simulink model "h"  (R2016a)
settings: Solver=VariableStepAuto  StartTime=0.0  StopTime=10.0  RelTol=1e-3
undefined symbols (not defined in the file): A, a1, a2, A3, A3A4, A4, b1, b2, beta, c1, c2, Cppx, Cppy, Cpx, Cpy, FM, Fs, M, m, R1, R2, R4, R5, RL, s, V4, V5, V5m, VA, VB, W_n1, yita_n1
settings Model: Creator=xlh  LastModifiedBy=xlh

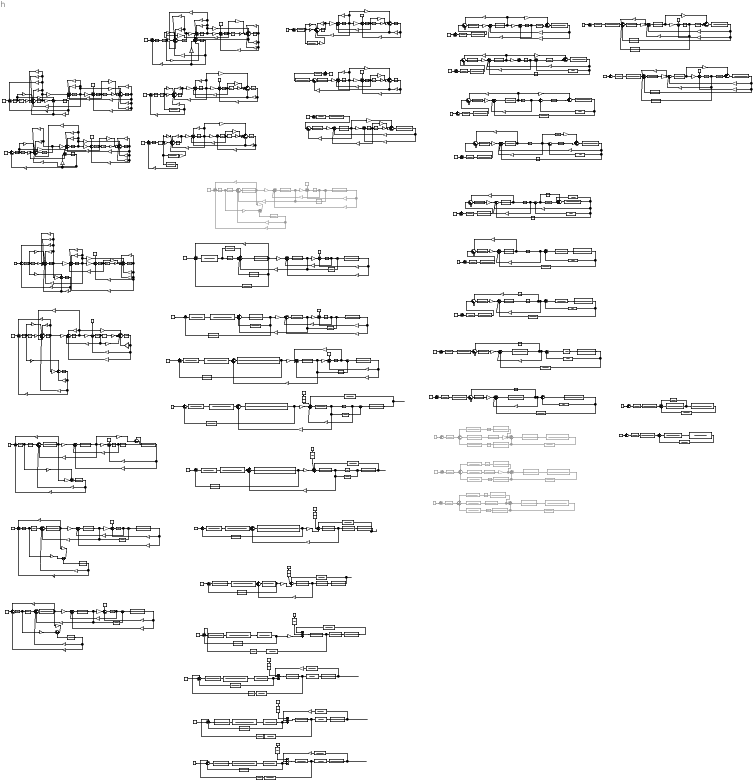
== system h ==
  note: 1.86e3rad/s
      | 296Hz
  note: 合并相同通道
  note: 合并相同通道
  note: y合并
  note: P4 合并
  note: V5-V4等式
  note: 忽略VB/beta
  note: 第三次化简P4
  note: 忽略, Cpx=3.3,远大于其他项，在频率为几赫兹时
  note: 忽略
  note: yita_n1=0.4725 W_n1=74081rad/s
  note: 第一次简化P5
  note: PB
  note: PB
  note: PB
  note: PB
  note: PB
  note: PB
  note: PB
  note: PB
  note: PB
  note: PB
  note: PB
  note: PB
  note: PB
  note: 第二次简化Vx
  note: PB
  note: 忽略
  note: yita_n1=0.4725 W_n1=74081rad/s
  note: PB
  note: 忽略
  note: yita_n1=0.4725 W_n1=74081rad/s
  note: PB
  note: 忽略, Cpx=3.3,远大于其他项，在频率为几赫兹时
  note: 忽略
  note: yita_n1=0.4725 W_n1=74081rad/s
  note: PB
  note: 忽略, Cpx=3.3,远大于其他项，在频率为几赫兹时
  note: 忽略
  note: yita_n1=0.4725 W_n1=74081rad/s
  note: PB
  note: PB
  note: PB
  note: PB
  note: PB
  note: PB
  note: PB
  note: 反馈通道合并
  note: PB
  note: x合并
  note: PB
  note: 挪动Vx',Vx'' = PA*A4/(Ms)-Vx'
  note: PB
  note: 合并
  note: PB
  note: x合并
  note: PB
  note: x合并
  note: PB
  note: Vx'''=-Vx''
  note: PB
  note: move branch
  note: PB
  note: merge
  note: PB
  note: move PB
  note: PB
  note: merge
  note: PB
  note: move
  note: PB
  note: simplify
  note: PB
  note: simplify
  note: PB
  note: move and merge
  note: PB
  note: 3.24e4rad/s
      | 5156Hz
      | 固定阻尼1.3747
  note: 1.86e3rad/s
      | 296Hz
  note: move
  note: PB
  note: 3.24e4rad/s
      | 5156Hz
      | 固定阻尼1.3747
  note: 合并相同通道
  note: desire frequent :1-10Hz
  note: move branch
  note: merge
  note: PB
  note: desire frequent :1-10Hz
  {1..5,8} (6 alike) : TransferFcn  Numerator=[A*R4*V5/beta (-Cpy*R4/V5)*beta -Cpy]  Denominator=[R4*V5/beta 1 0]
  {9..10,14..16,18..19,21,23..24,67..68} (12 alike) : Gain  Gain=1/R1
  17 : Gain  Gain=A4
  20 : Gain  Gain=A4
  6 : TransferFcn  Numerator=[A*R4*V5/beta (2*A+Cpy*R4*R5/beta) Cpy]  Denominator=[R4*V5/beta 1 0]
  7 : TransferFcn  Numerator=[A*R4*V5/beta (2*A+Cpy*R4*R5/beta) Cpy]  Denominator=[R4*V5/beta 1 0]
  95 : Gain  Gain=A4
  C3 : Constant  Value=Fs
  C4 : Constant  Value=Fs
  Constant{,2,4,6,8,10,14,16,18,20,22,24,26,28,30,32,34,36,38,40..42,44,46,48,50..59,64..65} (37 alike) : Constant  Value=FM
  Constant{1,3,5,7,9,11,15,17,19,21,23,25,27,29,31,33,35,37,39,43,45,47} (22 alike) : Constant  Value=Fs
  Constant{12,61..63} (4 alike) : Constant  Commented=on  Value=FM
  Constant13 : Constant  Commented=on  Value=Fs
  Gain{,20,44,142..143,165,193,208,229} (9 alike) : Gain  Gain=Cpy
  Gain{1,11..12,21,23..24,45,47..48,53,55,65,68,87,89,145,155,168,194,210} (20 alike) : Gain  Gain=1/R4
  Gain{10,22,144,209} (4 alike) : Gain  Gain=Cppy
  Gain100 : Gain  Commented=on  Gain=1/R4
  Gain101 : Gain  Commented=on  Gain=A4
  Gain{102,106,286..287} (4 alike) : Gain  Commented=on  Gain=1/R2
  Gain103 : Gain  Commented=on  Gain=A
  Gain104 : Gain  Commented=on  Gain=A3
  Gain105 : Gain  Commented=on  Gain=A
  Gain107 : Gain  Commented=on  Gain=A3
  Gain108 : Gain  Commented=on  Gain=A
  Gain109 : Gain  Commented=on  Gain=1/R1
  Gain{16,18,28,30,52,54,69,71,90,110,113,116,150,152,173..176,198..199,215,217,238..239,246..247} (26 alike) : Gain  Gain=A4
  Gain{2,7..8,14,26,32,37..38,56,61,70,72,76,84,91,95,111,114,118,120..121,125,129..132,134..138,148,154,159..161,177,182,185,190,195,200,204..205,213,219,223..225,240,244..245,249,254,261,265..267,270..271,273..274,276..277,279..280,282..283,285} (69 alike) : Gain  Gain=1/R2
  Gain{4,34,41,50,58,62,74,77,82,85,93,96,112,115,119,122..123,126,133,156,158,178,180..181,186,188..189,201,203,220,222,235,241,243,250,252..253,262..264,268..269,272,275,278,281,284,288} (48 alike) : Gain  Gain=A3
  Gain{13,15,25,27,42..43,66..67,80..81,88,98,117,127..128,147,149,192,212,214,231..234,248,255..258,260} (30 alike) : Gain  Gain=1/R1
  Gain{3,6,9,33,36,39..40,57,60,63..64,73,75,78..79,83,86,92,94,97,124,146,162,166,169,211,259} (27 alike) : Gain  Gain=A
  Gain139 : Gain  Gain=R2
  Gain140 : Gain  Gain=R2
  Gain141 : Gain  Gain=R2
  Gain{17,29,151,216} (4 alike) : Gain  Gain=1/RL
  Gain{19,31,153,218} (4 alike) : Gain  Gain=Cppx
  Gain{5,35,59,157,179,187,202,221,242,251} (10 alike) : Gain  Gain=Cpx
  Gain163 : Gain  Gain=2*A
  Gain164 : Gain  Gain=2/R4
  Gain{49,167,170,196,236} (5 alike) : Gain  Gain=1/R1+1/R2
  Gain{51,171..172,197,237} (5 alike) : Gain  Gain=1/R1+1/RL+Cppx
  Gain183 : Gain  Gain=1/R2+Cppy
  Gain{184,207,226,230} (4 alike) : Gain  Gain=A*s
  Gain191 : Gain  Gain=1/R2+Cppy
  Gain206 : Gain  Gain=1/R2+Cppy
  Gain227 : Gain  Gain=2*A*s
  Gain228 : Gain  Gain=2/R4
  Gain46 : Gain  Gain=Cppy+1/R4+1/R2
  Gain99 : Gain  Commented=on  Gain=1/R4
  Sum{,6,14,20,26,31,43,49,51,57..58,65,68,71..72,75,77,79,85,87,95,100,106,111,116,121,127,130,137,142,147,152,155,160,164,176..177} (37 alike) : Sum  Inputs=+--
  Sum{1,7,15,21,27,32,80,86,91,96,101} (11 alike) : Sum  Inputs=-----++
  Sum{4,10,12,18,24..25,42,47..48,83,89,93,98,104,109,114,119,126,135,140} (20 alike) : Sum  Inputs=--+
  Sum102 : Sum  Inputs=++-+
  Sum{3,9,17,23,29,34,45,52,55,82,88,92,97,103,108,113,118,134,139} (19 alike) : Sum  Inputs=--+++
  Sum{5,11,13,84,90,94,99,105,110,115,120,125,131,136,141,145} (16 alike) : Sum  Inputs=+-----
  Sum{64,107,112,117,122,128,143,148,153,157} (10 alike) : Sum  Inputs=|++
  Sum{123,129,144,149,154,158,162,166} (8 alike) : Sum  Inputs=--+-++
  Sum{67,70,73..74,76,78,124,163,178..180} (11 alike) : Sum  Inputs=+++
  Sum132 : Sum  Inputs=+-+
  Sum133 : Sum  Inputs=|++++
  Sum138 : Sum  Inputs=|++++
  Sum{30,35,46,53,56,61,146,151} (8 alike) : Sum  Inputs=|-+
  Sum150 : Sum  Inputs=------
  Sum156 : Sum  Inputs=+-+
  Sum{2,8,16,22,159} (5 alike) : Sum  Inputs=++-
  Sum161 : Sum  Inputs=|+-
  Sum165 : Sum  Inputs=|+-
  Sum{37,167..168,172} (4 alike) : Sum  Commented=on  Inputs=+--
  Sum{169..171,173..175} (6 alike) : Sum  Commented=on  Inputs=+++
  Sum19 : Sum  Inputs=+-
  Sum28 : Sum
  Sum33 : Sum
  Sum36 : Sum  Commented=on  Inputs=--+
  Sum38 : Sum  Commented=on  Inputs=-----++
  Sum39 : Sum  Commented=on
  Sum40 : Sum  Commented=on  Inputs=--+++
  Sum41 : Sum  Commented=on  Inputs=|-+
  Sum{44,54,59,62,66,69} (6 alike) : Sum  Inputs=+--+-++
  Sum50 : Sum  Inputs=+----++
  Sum60 : Sum  Inputs=+++++
  Sum63 : Sum  Inputs=+++++
  Sum81 : Sum  Inputs=++-+
  T1 : TransferFcn  Numerator=[M 0]  Denominator=[A3*R2]
  Tra : TransferFcn  Numerator=[beta]  Denominator=[V4 0]
  Transfer Fcn{,8,22,30,38,45,149,157,165,183} (10 alike) : TransferFcn  Denominator=[m 0]
  Transfer Fcn{1,7,9,15,21,23,150,156,158,164,166,172,181,184,190,194,201} (17 alike) : TransferFcn  Denominator=[1 0]
  Transfer Fcn{2,10,16,159,167,176,185} (7 alike) : TransferFcn  Numerator=[beta]  Denominator=[V4 0]
  Transfer Fcn{88,100,103,113} (4 alike) : TransferFcn  Denominator=[(VB/beta+M) 1/R1+1/R2]
  Transfer Fcn{35,43,59,69,78,86,93,101,107,114} (10 alike) : TransferFcn  Numerator=[A4 Cpx]  Denominator="[VA/beta  (1/R1+1/RL+Cppx) 0]"
  Transfer Fcn102 : TransferFcn  Numerator="[A3A4  (M/R1+A3*Cpx)]"  Denominator=[A4*M M*Cpx 0]
  Transfer Fcn{64,71,82,90,96,104} (6 alike) : TransferFcn  Numerator=[V5/beta 1/R4]  Denominator=[V5m/beta m/R4 A^2]
  Transfer Fcn{91,97,105,110,117,126,135,144,151,268,272,280,286,323,326} (15 alike) : TransferFcn  Numerator=[M/R1 A3*A4]  Denominator=[M 0]
  Transfer Fcn{6,14,20,28,36,44,60,70,79,92,98,106,111,118,155,163,171,180,189,193,200,206,211,227,235} (25 alike) : TransferFcn  Denominator=[M 0]
  Transfer Fcn108 : TransferFcn  Numerator="[A3A4  (M/R1+A3*Cpx)]"  Denominator=[A4*M M*Cpx 0]
  Transfer Fcn{109,116,125,134,143} (5 alike) : TransferFcn  Numerator=[1/m beta/(R4*V5*m)]  Denominator=[1 2*yita_n1*W_n1 W_n1^2]
  Transfer Fcn{3,11,17,152,186} (5 alike) : TransferFcn  Numerator=[beta]  Denominator=[V5 0]
  Transfer Fcn{57,76,83..84,99,112,119,128,137,146} (10 alike) : TransferFcn  Numerator=[-A*R4*V5/beta 0]  Denominator=[R4*V5/beta 1]
  Transfer Fcn115 : TransferFcn  Numerator="[A3A4  (M/R1+A3*Cpx)]"  Denominator=[A4*M M*Cpx 0]
  Transfer Fcn{4,12,18,153,161,169,178,187,191} (9 alike) : TransferFcn  Numerator=[beta]  Denominator=[VB 0]
  Transfer Fcn{120,129,138,147} (4 alike) : TransferFcn  Numerator=[A*beta^2 0]  Denominator=[R4*V5 beta]
  Transfer Fcn{121,130,139,148} (4 alike) : TransferFcn  Denominator=[R2*V4 0]
  Transfer Fcn122 : TransferFcn  Denominator=[(VB/beta+M)*R2 R2/R1+1]
  Transfer Fcn123 : TransferFcn  Numerator=[Cpx]  Denominator="[VA/beta  (1/R1+1/RL+Cppx) 0]"
  Transfer Fcn124 : TransferFcn  Numerator=[(A3*Cpx)]  Denominator=[M*Cpx 0]
  Transfer Fcn127 : TransferFcn  Numerator=[R2]  Denominator=[M 0]
  Transfer Fcn{5,13,19,154,162,170,179,188,192} (9 alike) : TransferFcn  Numerator=[beta]  Denominator=[VA 0]
  Transfer Fcn131 : TransferFcn  Denominator=[M*R2 R2/R1+1]
  Transfer Fcn132 : TransferFcn  Numerator=[Cpx]  Denominator="[VA/beta  (1/R1+1/RL+Cppx) 0]"
  Transfer Fcn133 : TransferFcn  Numerator=[(A3*Cpx)]  Denominator=[M*Cpx 0]
  Transfer Fcn136 : TransferFcn  Numerator=[R2]  Denominator=[M 0]
  Transfer Fcn140 : TransferFcn  Denominator=[(VB/beta+M)*R2 R2/R1+1]
  Transfer Fcn141 : TransferFcn  Numerator=[Cpx]  Denominator="[VA/beta  (1/R1+1/RL+Cppx) 0]"
  Transfer Fcn142 : TransferFcn  Numerator=[(A3*Cpx)]  Denominator=[M*Cpx 0]
  Transfer Fcn145 : TransferFcn  Numerator=[R2]  Denominator=[M 0]
  Transfer Fcn{160,168,173,182} (4 alike) : TransferFcn  Numerator=[2*A Cpy]  Denominator=[V5/beta 2/R4]
  Transfer Fcn174 : TransferFcn  Denominator=[a1 b1 c1]
  Transfer Fcn175 : TransferFcn  Denominator=[a1 b1 c1]
  Transfer Fcn{177,197,199,204,217,223..225,233,241,250,261,274} (13 alike) : TransferFcn  Denominator=[V4/beta 1/R2+Cppy]
  Transfer Fcn{195,202,208,213,221,229,237,245,254,265,270,278,284} (13 alike) : TransferFcn  Numerator=[-V5*A/beta/R4 2*A Cpy]  Denominator=[V5/beta/R4 2/R4^2]
  Transfer Fcn196 : TransferFcn  Denominator=[a1 b1 c1]
  Transfer Fcn{27,198,205,210,218,226,234,242,251} (9 alike) : TransferFcn  Denominator=[VA/beta 1/R1+1/RL+Cppx]
  Transfer Fcn{26,34,42,58,68,77,85,203,209,214,222,230,238,246,255,266,271} (17 alike) : TransferFcn  Denominator=[VB/beta 1/R1+1/R2]
  Transfer Fcn{29,207,212,220,228,236,244,253} (8 alike) : TransferFcn  Numerator=[A4 Cpx]  Denominator=[1 0]
  Transfer Fcn{215,256,259..260,327,329..330,332} (8 alike) : TransferFcn  Numerator=[A4]  Denominator=[M 0]
  Transfer Fcn216 : TransferFcn  Numerator=[A3*A4]  Denominator=[M 0]
  Transfer Fcn{94,219,243,252,263,267} (6 alike) : TransferFcn  Numerator=[A3]  Denominator=[M 0]
  Transfer Fcn231 : TransferFcn  Numerator=[A3/R2]  Denominator=[VB/beta 1/R1+1/R2]
  Transfer Fcn232 : TransferFcn  Numerator=[1/R2*R1]  Denominator=[VB/beta 1/R1+1/R2]
  Transfer Fcn239 : TransferFcn  Numerator=[A3/R2]  Denominator=[VB/beta 1/R1+1/R2]
  Transfer Fcn{24,32,37,56,66} (5 alike) : TransferFcn  Denominator=[V4/beta Cppy+1/R4+1/R2]
  Transfer Fcn240 : TransferFcn  Numerator=[1/R2*R1]  Denominator=[VB/beta 1/R1+1/R2]
  Transfer Fcn247 : TransferFcn  Denominator=[(VA/beta) 1/R1+1/RL+Cppx+A4/A3/R1]
  Transfer Fcn248 : TransferFcn  Numerator=[A3*A4]  Denominator=[M 0]
  Transfer Fcn249 : TransferFcn  Numerator=[M 0]  Denominator=[A3]
  Transfer Fcn25 : TransferFcn  Denominator=[V5/beta 1/R4]
  Transfer Fcn257 : TransferFcn  Numerator=[A3*A4]  Denominator=[M 0]
  Transfer Fcn258 : TransferFcn  Numerator=[M 0]  Denominator=[A3*R1]
  Transfer Fcn262 : TransferFcn  Denominator=[(VA/beta) 1/R1+1/RL+Cppx+A4/A3/R1]
  Transfer Fcn264 : TransferFcn  Numerator=[-M/A3/R1 -A4 -Cpx]  Denominator=[1 0]
  Transfer Fcn269 : TransferFcn  Numerator=[M/A3/R1 A4 Cpx]  Denominator=[1 0]
  Transfer Fcn273 : TransferFcn  Numerator=[M 0]  Denominator=[A3]
  Transfer Fcn275 : TransferFcn  Denominator=[(VA/beta) 1/R1+1/RL+Cppx+A4/A3/R1]
  Transfer Fcn276 : TransferFcn  Numerator=[Cpx]  Denominator=[(VA/beta) 1/R1+1/RL+Cppx+A4/A3/R1 0]
  Transfer Fcn277 : TransferFcn  Numerator=[Cpx]  Denominator=[1 0]
  Transfer Fcn279 : TransferFcn  Numerator=[A3]  Denominator=[M*VB/beta M/R1+M/R2 0]
  Transfer Fcn281 : TransferFcn  Numerator=[M 0]  Denominator=[A3*R2]
  Transfer Fcn283 : TransferFcn  Commented=on  Denominator=[V4/beta 1/R2+Cppy]
  Transfer Fcn285 : TransferFcn  Numerator=[A3]  Denominator=[M*VB/beta M/R1+M/R2 0]
  Transfer Fcn287 : TransferFcn  Numerator=[-M/A3/R1 -A4 -Cpx]  Denominator=[(VA/beta) A4^2 Cpx*A4]
  Transfer Fcn288 : TransferFcn  Commented=on  Numerator=[M/A3/R1 A4 Cpx]  Denominator=[(VA/beta+2*M*A4/A3/R1) A4^2 Cpx*A4]
  Transfer Fcn289 : TransferFcn  Commented=on  Numerator=[-V5*A/beta/R4 2*A Cpy]  Denominator=[V5/beta/R4 2/R4^2]
  Transfer Fcn290 : TransferFcn  Commented=on  Numerator=[A3]  Denominator=[M*VB/beta M/R1+M/R2 A3^2]
  Transfer Fcn291 : TransferFcn  Commented=on  Numerator=[M/R1 A3*A4]  Denominator=[M 0]
  Transfer Fcn{292,294,301,303,314,316} (6 alike) : TransferFcn  Commented=on  Numerator=[M 0]  Denominator=[A3*R2]
  Transfer Fcn{293,295,302,304,315,317} (6 alike) : TransferFcn  Commented=on  Numerator=[M*VB/beta M/R1+M/R2 A3^2]  Denominator=[A3]
  Transfer Fcn296 : TransferFcn  Commented=on  Denominator=[V4/beta 1/R2+Cppy]
  Transfer Fcn297 : TransferFcn  Commented=on  Numerator=[M/A3/R1 A4 Cpx]  Denominator=[(VA/beta+2*M*A4/A3/R1) A4^2 Cpx*A4]
  Transfer Fcn298 : TransferFcn  Commented=on  Numerator=[ 2*A Cpy]  Denominator=[V5/beta/R4 2/R4^2]
  Transfer Fcn299 : TransferFcn  Commented=on  Numerator=[A3]  Denominator=[M*VB/beta M/R1+M/R2 A3^2]
  Transfer Fcn300 : TransferFcn  Commented=on  Numerator=[M/R1 A3*A4]  Denominator=[M 0]
  Transfer Fcn305 : TransferFcn  Commented=on  Numerator=[V5/beta/R4 2/R4^2]  Denominator=[-V5*A/beta/R4 2*A Cpy]
  Transfer Fcn306 : TransferFcn  Commented=on  Numerator=[V5/beta/R4 2/R4^2]  Denominator=[-V5*A/beta/R4 2*A Cpy]
  Transfer Fcn{307..308,318..319} (4 alike) : TransferFcn  Commented=on  Numerator=[V5/beta/R4 2/R4^2]  Denominator=[2*A Cpy]
  Transfer Fcn309 : TransferFcn  Commented=on  Denominator=[V4*R2/beta 1+Cppy*R2]
  Transfer Fcn{31,39,46,72} (4 alike) : TransferFcn  Numerator=[A Cpy]  Denominator=[1 0]
  Transfer Fcn310 : TransferFcn  Commented=on  Numerator=[M/A3/R1 A4 Cpx]  Denominator=[(VA/beta+2*M*A4/A3/R1) A4^2 Cpx*A4]
  Transfer Fcn311 : TransferFcn  Commented=on  Numerator=[ 2*A Cpy]  Denominator=[V5/beta/R4 2/R4^2]
  Transfer Fcn312 : TransferFcn  Commented=on  Numerator=[A3]  Denominator=[M*VB/beta M/R1+M/R2 A3^2]
  Transfer Fcn313 : TransferFcn  Commented=on  Numerator=[M/R1 A3*A4]  Denominator=[M 0]
  Transfer Fcn320 : TransferFcn  Numerator=[M/A3/R1 A4 Cpx]  Denominator=[(VA/beta+2*M*A4/A3/R1) A4^2 Cpx*A4]
  Transfer Fcn321 : TransferFcn  Numerator=[-V5*A/beta/R4 2*A Cpy]  Denominator=[a2 b2 c2]
  Transfer Fcn322 : TransferFcn  Numerator=[A3]  Denominator=[M*VB/beta (M/R1+M/R2) A3^2]
  Transfer Fcn324 : TransferFcn  Numerator=[-V5*A/beta/R4 2*A Cpy]  Denominator=[a2 b2 c2]
  Transfer Fcn325 : TransferFcn  Numerator=[A3]  Denominator=[M*VB/beta (M/R1) A3^2]
  Transfer Fcn328 : TransferFcn  Numerator=[A4]  Denominator=[A3*R1]
  Transfer Fcn33 : TransferFcn  Denominator=[V5/beta 1/R4]
  Transfer Fcn331 : TransferFcn  Numerator=[M 0]  Denominator=[A3*R2]
  Transfer Fcn40 : TransferFcn  Denominator=[V5/beta 1/R4]
  Transfer Fcn{41,47,63,73,81,89,95} (7 alike) : TransferFcn  Numerator=[1/R1 0]  Denominator=[A4 Cpx]
  Transfer Fcn48 : TransferFcn  Commented=on  Denominator=[V4/beta Cppy+1/R4+1/R2]
  Transfer Fcn49 : TransferFcn  Commented=on  Denominator=[V5/beta 1/R4]
  Transfer Fcn50 : TransferFcn  Commented=on  Denominator=[VB/beta 1/R1+1/R2]
  Transfer Fcn51 : TransferFcn  Commented=on  Numerator=[A4 Cpx]  Denominator="[VA/beta  (1/R1+1/RL+Cppx) 0]"
  Transfer Fcn52 : TransferFcn  Commented=on  Denominator=[M 0]
  Transfer Fcn53 : TransferFcn  Commented=on  Denominator=[m 0]
  Transfer Fcn54 : TransferFcn  Commented=on  Numerator=[A Cpy]  Denominator=[1 0]
  Transfer Fcn55 : TransferFcn  Commented=on  Numerator=[1/R1 0]  Denominator=[A4 Cpx]
  Transfer Fcn61 : TransferFcn  Numerator="[R4^2*V5/beta  R4]"  Denominator="[V4*R4^2*V5/beta^2  ((Cppy+1/R4+1/R2)*R4^2*V5/beta+R4*V4/beta) R4*Cppy+R4/R2]"
  Transfer Fcn62 : TransferFcn  Numerator=[A*R4*V5/beta (-Cpy*R4/V5)*beta -Cpy]  Denominator=[R4*V5/beta 1 0]
  Transfer Fcn65 : TransferFcn  Denominator=[R4^2*V5/beta R4]
  Transfer Fcn67 : TransferFcn  Numerator=[A]  Denominator=[R4*V5/beta 1]
  Transfer Fcn74 : TransferFcn  Numerator=[A]  Denominator=[R4*V5/beta 1]
  Transfer Fcn75 : TransferFcn  Denominator=[R4^2*V5/beta R4]
  Transfer Fcn80 : TransferFcn  Numerator=[A*R4*V5/beta (-Cpy*R4/V5)*beta -Cpy]  Denominator=[R4*V5/beta 1 0]
  Transfer Fcn87 : TransferFcn  Numerator=[-A3]  Denominator=[M 0]
  a1 : TransferFcn  Numerator="[R4^2*V5/beta  R4]"  Denominator="[V4*R4^2*V5/beta^2  ((Cppy+1/R4+1/R2)*R4^2*V5/beta+R4*V4/beta) R4*Cppy+R4/R2]"
  a2 : TransferFcn  Numerator="[R4*V5/beta  1]"  Denominator="[V4*R4^2*V5/beta^2  ((Cppy+1/R4+1/R2)*R4^2*V5/beta+R4*V4/beta) R4*Cppy+R4/R2]"
  a3 : TransferFcn  Numerator="[R4^2*V5/beta  R4]"  Denominator="[V4*R4^2*V5/beta^2  ((Cppy+1/R4+1/R2)*R4^2*V5/beta+R4*V4/beta) R4*Cppy+R4/R2]"
  a{4..8} (5 alike) : TransferFcn  Numerator=[beta^2/(V4*R4*V5)]  Denominator="[1  0 0]"
  先导级{,1..10,14..15} (13 alike) : TransferFcn  Denominator=[a1 b1 c1]
  先导级11 : TransferFcn  Commented=on  Denominator=[a1 b1 c1]
  先导级12 : TransferFcn  Commented=on  Denominator=[a1 b1 c1]
  先导级13 : TransferFcn  Commented=on  Denominator=[a1 b1 c1]
  wires:
  Sum/1 -> Transfer Fcn/1
  Transfer Fcn/1 -> Gain9/1, Gain259/1, Transfer Fcn1/1  "Vy"
  Transfer Fcn1/1 -> Gain/1  "y"
  Gain/1 -> Sum1/4
  Constant/1 -> Sum/2
  Sum1/1 -> Transfer Fcn2/1
  Transfer Fcn2/1 -> Gain11/1, Gain10/1, Gain6/1, Gain8/1, Gain2/1, Gain1/1  "P4"
  Gain1/1 -> Sum2/2
  Sum2/1 -> Transfer Fcn3/1
  Transfer Fcn3/1 -> Gain12/1, Gain3/1  "P5"
  Gain3/1 -> Sum/3
  Gain2/1 -> Sum3/3
  Sum3/1 -> Transfer Fcn4/1
  Transfer Fcn4/1 -> Gain257/1, Gain14/1, Gain13/1, Gain7/1, Gain4/1
  Gain4/1 -> Sum4/2
  Sum4/1 -> Transfer Fcn6/1
  Transfer Fcn6/1 -> Gain50/1, Gain18/1, Transfer Fcn7/1  "Vx"
  Transfer Fcn7/1 -> Gain5/1  "x"
  Gain5/1 -> Sum5/4
  Sum5/1 -> Transfer Fcn5/1
  Transfer Fcn5/1 -> Gain16/1, Gain17/1, Gain15/1, Gain256/1, Gain19/1  "PA"
  Gain6/1 -> Sum/1
  Gain7/1 -> Sum1/7
  Gain8/1 -> Sum1/1
  Gain9/1 -> Sum1/2
  Gain10/1 -> Sum1/3
  Gain11/1 -> Sum1/5
  Gain12/1 -> Sum1/6, Sum2/3
  Gain13/1 -> Sum3/1
  Gain14/1 -> Sum3/2
  Gain15/1 -> Sum5/6
  Constant1/1 -> Sum4/1
  Gain16/1 -> Sum4/3
  Gain17/1 -> Sum5/5
  Gain18/1 -> Sum5/3
  Gain19/1 -> Sum5/2
  Sum6/1 -> Transfer Fcn8/1
  Transfer Fcn8/1 -> Gain40/1, Gain39/1, Transfer Fcn9/1  "Vy"
  Transfer Fcn9/1 -> Gain20/1  "y"
  Gain20/1 -> Sum7/4
  Constant2/1 -> Sum6/2
  Sum7/1 -> Transfer Fcn10/1
  Transfer Fcn10/1 -> Gain23/1, Gain22/1, Gain36/1, Gain38/1, Gain21/1, Gain32/1  "P4"
  Gain21/1 -> Sum8/2
  Sum8/1 -> Transfer Fcn11/1
  Transfer Fcn11/1 -> Gain24/1, Gain33/1  "P5"
  Gain33/1 -> Sum6/3
  Gain32/1 -> Sum9/3
  Sum9/1 -> Transfer Fcn12/1
  Transfer Fcn12/1 -> Gain42/1, Gain26/1, Gain25/1, Gain37/1, Gain34/1
  Gain34/1 -> Sum10/2
  Sum10/1 -> Transfer Fcn14/1
  Transfer Fcn14/1 -> Gain41/1, Gain30/1, Transfer Fcn15/1  "Vx"
  Transfer Fcn15/1 -> Gain35/1  "x"
  Gain35/1 -> Sum11/4
  Sum11/1 -> Transfer Fcn13/1
  Transfer Fcn13/1 -> Gain43/1, Gain28/1, Gain29/1, Gain27/1, Gain31/1  "PA"
  Gain36/1 -> Sum6/1
  Gain37/1 -> Sum7/7
  Gain38/1 -> Sum7/1
  Gain39/1 -> Sum7/2
  Gain22/1 -> Sum7/3
  Gain23/1 -> Sum7/5
  Gain24/1 -> Sum7/6, Sum8/3
  Gain25/1 -> Sum9/1
  Gain26/1 -> Sum9/2
  Gain27/1 -> Sum11/6
  Constant3/1 -> Sum10/1
  Gain28/1 -> Sum10/3
  Gain29/1 -> Sum11/5
  Gain30/1 -> Sum11/3
  Gain31/1 -> Sum11/2
  Gain40/1 -> Sum8/1
  Gain42/1 -> Sum11/1
  Gain43/1 -> Sum9/5
  Sum14/1 -> Transfer Fcn22/1
  Transfer Fcn22/1 -> Gain64/1, Gain63/1, Transfer Fcn23/1  "Vy"
  Transfer Fcn23/1 -> Gain44/1  "y"
  Gain44/1 -> Sum15/4
  Constant4/1 -> Sum14/2
  Sum15/1 -> Transfer Fcn16/1
  Transfer Fcn16/1 -> Gain60/1, Gain46/1, Gain45/1, Gain56/1  "P4"
  Gain45/1 -> Sum16/2
  Sum16/1 -> Transfer Fcn17/1
  Transfer Fcn17/1 -> Gain47/1, Gain57/1, Gain48/1  "P5"
  Gain57/1 -> Sum14/3
  Gain56/1 -> Sum17/3
  Sum17/1 -> Transfer Fcn18/1
  Transfer Fcn18/1 -> Gain61/1, Gain66/1, Gain49/1, Gain58/1
  Gain58/1 -> Sum12/2
  Sum12/1 -> Transfer Fcn20/1
  Transfer Fcn20/1 -> Gain62/1, Gain54/1, Transfer Fcn21/1  "Vx"
  Transfer Fcn21/1 -> Gain59/1  "x"
  Gain59/1 -> Sum13/4
  Sum13/1 -> Transfer Fcn19/1
  Transfer Fcn19/1 -> Gain67/1, Gain52/1, Gain51/1  "PA"
  Gain60/1 -> Sum14/1
  Gain61/1 -> Sum15/7
  Gain63/1 -> Sum15/2
  Gain48/1 -> Sum16/3
  Gain49/1 -> Sum17/1
  Gain51/1 -> Sum13/6
  Constant5/1 -> Sum12/1
  Gain52/1 -> Sum12/3
  Gain64/1 -> Sum16/1
  Gain66/1 -> Sum13/1
  Gain67/1 -> Sum17/5
  Gain47/1 -> Sum15/6
  Gain50/1 -> Sum3/4
  Gain62/1 -> Sum17/4
  Gain41/1 -> Sum9/4
  Gain54/1 -> Sum13/5
  Gain46/1 -> Sum15/1
  Sum20/1 -> Transfer Fcn30/1
  Transfer Fcn30/1 -> Transfer Fcn31/1, Gain79/1  "Vy"
  Transfer Fcn31/1 -> Sum21/4
  Constant6/1 -> Sum20/2
  Sum21/1 -> Transfer Fcn24/1
  Transfer Fcn24/1 -> Gain55/1, Gain75/1, Gain72/1  "P4"
  Gain55/1 -> Sum22/2
  Sum22/1 -> Transfer Fcn25/1
  Transfer Fcn25/1 -> Gain73/1, Gain68/1  "P5"
  Gain73/1 -> Sum20/3
  Gain72/1 -> Sum23/3
  Sum23/1 -> Transfer Fcn26/1
  Transfer Fcn26/1 -> Gain80/1, Gain76/1, Gain74/1
  Gain74/1 -> Sum18/2
  Sum18/1 -> Transfer Fcn28/1
  Transfer Fcn28/1 -> Gain77/1, Transfer Fcn29/1  "Vx"
  Transfer Fcn29/1 -> Sum19/2
  Sum19/1 -> Transfer Fcn27/1
  Transfer Fcn27/1 -> Gain71/1, Gain81/1  "PA"
  Gain75/1 -> Sum20/1
  Gain76/1 -> Sum21/7
  Constant7/1 -> Sum18/1
  Gain71/1 -> Sum18/3
  Gain79/1 -> Sum22/1
  Gain80/1 -> Sum19/1
  Gain81/1 -> Sum23/5
  Gain68/1 -> Sum21/6
  Gain77/1 -> Sum23/4
  Sum26/1 -> Transfer Fcn38/1
  Transfer Fcn38/1 -> Gain86/1, Transfer Fcn39/1  "Vy"
  Transfer Fcn39/1 -> Sum27/4
  Constant8/1 -> Sum26/2
  Sum27/1 -> Transfer Fcn32/1
  Transfer Fcn32/1 -> Gain53/1, Gain83/1, Gain70/1  "P4"
  Gain53/1 -> Sum28/2
  Sum28/1 -> Transfer Fcn33/1
  Transfer Fcn33/1 -> Gain78/1, Gain65/1  "P5"
  Gain78/1 -> Sum26/3
  Gain70/1 -> Sum29/3
  Sum29/1 -> Transfer Fcn34/1
  Transfer Fcn34/1 -> Gain84/1, Transfer Fcn41/1, Gain82/1
  Gain82/1 -> Sum24/2
  Sum24/1 -> Transfer Fcn36/1
  Transfer Fcn36/1 -> Sum30/1, Gain85/1  "Vx"
  Transfer Fcn35/1 -> Gain88/1, Gain69/1  "PA"
  Gain83/1 -> Sum26/1
  Gain84/1 -> Sum27/7
  Constant9/1 -> Sum24/1
  Gain69/1 -> Sum24/3
  Gain86/1 -> Sum28/1
  Gain88/1 -> Sum29/5
  Gain65/1 -> Sum27/6
  Gain85/1 -> Sum29/4
  Transfer Fcn41/1 -> Sum30/2
  Sum30/1 -> Transfer Fcn35/1
  Sum31/1 -> Transfer Fcn45/1
  Transfer Fcn45/1 -> Gain97/1, Transfer Fcn46/1  "Vy"
  Transfer Fcn46/1 -> Sum32/4
  Constant10/1 -> Sum31/2
  Sum32/1 -> Transfer Fcn37/1
  Transfer Fcn37/1 -> Gain87/1, Gain94/1, Gain91/1  "P4"
  Gain87/1 -> Sum33/2
  Sum33/1 -> Transfer Fcn40/1
  Transfer Fcn40/1 -> Gain92/1, Gain89/1  "P5"
  Gain92/1 -> Sum31/3
  Gain91/1 -> Sum34/3
  Sum34/1 -> Transfer Fcn42/1
  Transfer Fcn42/1 -> Gain95/1, Transfer Fcn47/1, Gain93/1
  Gain93/1 -> Sum25/2
  Sum25/1 -> Transfer Fcn44/1
  Transfer Fcn44/1 -> Sum35/1, Gain96/1  "Vx"
  Transfer Fcn43/1 -> Gain98/1, Gain90/1  "PA"
  Gain94/1 -> Sum31/1
  Gain95/1 -> Sum32/7
  Constant11/1 -> Sum25/1
  Gain90/1 -> Sum25/3
  Gain97/1 -> Sum33/1
  Gain98/1 -> Sum34/5
  Gain89/1 -> Sum32/6
  Gain96/1 -> Sum34/4
  Transfer Fcn47/1 -> Sum35/2
  Sum35/1 -> Transfer Fcn43/1
  Sum37/1 -> Transfer Fcn53/1
  Transfer Fcn53/1 -> Gain108/1, Transfer Fcn54/1  "Vy"
  Transfer Fcn54/1 -> Sum38/4
  Constant12/1 -> Sum37/2
  Sum38/1 -> Transfer Fcn48/1
  Transfer Fcn48/1 -> Gain99/1, Gain105/1, Gain102/1  "P4"
  Gain99/1 -> Sum39/2
  Sum39/1 -> Transfer Fcn49/1
  Transfer Fcn49/1 -> Gain103/1, Gain100/1  "P5"
  Gain103/1 -> Sum37/3
  Gain102/1 -> Sum40/3
  Sum40/1 -> Transfer Fcn50/1
  Transfer Fcn50/1 -> Gain106/1, Transfer Fcn55/1, Gain104/1
  Gain104/1 -> Sum36/2
  Sum36/1 -> Transfer Fcn52/1
  Transfer Fcn52/1 -> Sum41/1, Gain107/1  "Vx"
  Transfer Fcn51/1 -> Gain109/1, Gain101/1  "PA"
  Gain105/1 -> Sum37/1
  Gain106/1 -> Sum38/7
  Constant13/1 -> Sum36/1
  Gain101/1 -> Sum36/3
  Gain108/1 -> Sum39/1
  Gain109/1 -> Sum40/5
  Gain100/1 -> Sum38/6
  Gain107/1 -> Sum40/4
  Transfer Fcn55/1 -> Sum41/2
  Sum41/1 -> Transfer Fcn51/1
  Sum49/1 -> Transfer Fcn71/1
  Transfer Fcn71/1 -> Transfer Fcn72/1, Transfer Fcn74/1  "Vy"
  Transfer Fcn72/1 -> Sum50/4
  Constant16/1 -> Sum49/2
  Sum50/1 -> Transfer Fcn66/1
  Transfer Fcn66/1 -> Transfer Fcn67/1, Transfer Fcn75/1, Gain124/1, Gain121/1  "P4"
  Transfer Fcn67/1 -> Sum49/3  "P5'"
  Gain121/1 -> Sum52/3
  Sum52/1 -> Transfer Fcn68/1
  Transfer Fcn68/1 -> Gain125/1, Transfer Fcn73/1, Gain123/1
  Gain123/1 -> Sum48/2
  Sum48/1 -> Transfer Fcn70/1
  Transfer Fcn70/1 -> Sum53/1, Gain126/1  "Vx"
  Transfer Fcn69/1 -> Gain128/1, Gain116/1  "PA"
  Gain124/1 -> Sum49/1
  Gain125/1 -> Sum50/7
  Constant17/1 -> Sum48/1
  Gain116/1 -> Sum48/3
  Gain128/1 -> Sum52/5
  Transfer Fcn75/1 -> Sum50/6
  Gain126/1 -> Sum52/4
  Transfer Fcn73/1 -> Sum53/2
  Sum53/1 -> Transfer Fcn69/1
  Transfer Fcn74/1 -> Sum50/1
  Sum43/1 -> Transfer Fcn64/1
  Transfer Fcn64/1 -> Transfer Fcn62/1  "Vy"
  Transfer Fcn62/1 -> Sum44/4
  Constant14/1 -> Sum43/2
  Sum44/1 -> Transfer Fcn56/1
  Transfer Fcn56/1 -> Transfer Fcn57/1, Transfer Fcn65/1, Gain111/1  "P4"
  Transfer Fcn57/1 -> Sum43/3  "P5'"
  Gain111/1 -> Sum45/3
  Sum45/1 -> Transfer Fcn58/1
  Transfer Fcn58/1 -> Gain114/1, Transfer Fcn63/1, Gain112/1
  Gain112/1 -> Sum42/2
  Sum42/1 -> Transfer Fcn60/1
  Transfer Fcn60/1 -> Sum46/1, Gain115/1  "Vx"
  Transfer Fcn59/1 -> Gain117/1, Gain110/1  "PA"
  Gain114/1 -> Sum44/7
  Constant15/1 -> Sum42/1
  Gain110/1 -> Sum42/3
  Gain117/1 -> Sum45/5
  Transfer Fcn65/1 -> Sum44/6
  Gain115/1 -> Sum45/4
  Transfer Fcn63/1 -> Sum46/2
  Sum46/1 -> Transfer Fcn59/1
  Sum51/1 -> Transfer Fcn82/1
  Transfer Fcn82/1 -> Transfer Fcn80/1  "Vy"
  Transfer Fcn80/1 -> Sum54/4
  Constant18/1 -> Sum51/2
  Sum54/1 -> Transfer Fcn61/1
  Transfer Fcn61/1 -> Gain118/1, Transfer Fcn76/1  "P4"
  Transfer Fcn76/1 -> Sum51/3  "P5'"
  Gain118/1 -> Sum55/3
  Sum55/1 -> Transfer Fcn77/1
  Transfer Fcn77/1 -> Gain120/1, Transfer Fcn81/1, Gain119/1
  Gain119/1 -> Sum47/2
  Sum47/1 -> Transfer Fcn79/1
  Transfer Fcn79/1 -> Sum56/1, Gain122/1  "Vx"
  Transfer Fcn78/1 -> Gain127/1, Gain113/1  "PA"
  Gain120/1 -> Sum54/7
  Constant19/1 -> Sum47/1
  Gain113/1 -> Sum47/3
  Gain127/1 -> Sum55/5
  Gain122/1 -> Sum55/4
  Transfer Fcn81/1 -> Sum56/2
  Sum56/1 -> Transfer Fcn78/1
  Sum58/1 -> Transfer Fcn90/1
  Transfer Fcn90/1 -> 8/1  "Vy"
  8/1 -> Sum59/4
  Constant20/1 -> Sum58/2
  Sum59/1 -> a3/1
  a3/1 -> Gain130/1, Transfer Fcn84/1  "P4"
  Transfer Fcn84/1 -> Sum58/3  "P5'"
  Gain130/1 -> Sum60/3
  Sum60/1 -> Transfer Fcn85/1
  Transfer Fcn85/1 -> Transfer Fcn87/1, Gain132/1, Transfer Fcn89/1
  Transfer Fcn87/1 -> Sum61/1, Gain133/1  "Vx'"
  Transfer Fcn86/1 -> Transfer Fcn91/1  "PA"
  Gain132/1 -> Sum59/7
  Gain133/1 -> Sum60/4
  Transfer Fcn89/1 -> Sum61/2
  Sum61/1 -> Transfer Fcn86/1
  Transfer Fcn91/1 -> Sum60/1
  Constant21/1 -> Transfer Fcn92/1
  Transfer Fcn92/1 -> Sum60/2
  Sum57/1 -> Transfer Fcn96/1
  Transfer Fcn96/1 -> 1/1  "Vy"
  1/1 -> Sum62/4
  Constant22/1 -> Sum57/2
  Sum62/1 -> a1/1
  a1/1 -> Gain129/1, Transfer Fcn83/1  "P4"
  Transfer Fcn83/1 -> Sum57/3  "P5'"
  Gain129/1 -> Sum63/3
  Sum63/1 -> Transfer Fcn88/1
  Transfer Fcn88/1 -> Transfer Fcn94/1, Gain131/1, Transfer Fcn95/1
  Transfer Fcn94/1 -> Sum64/1  "Vx'"
  Transfer Fcn93/1 -> Transfer Fcn97/1  "PA"
  Gain131/1 -> Sum62/7
  Transfer Fcn95/1 -> Sum64/2
  Sum64/1 -> Transfer Fcn93/1
  Transfer Fcn97/1 -> Sum63/1
  Constant23/1 -> Transfer Fcn98/1
  Transfer Fcn98/1 -> Sum63/2
  Sum65/1 -> Transfer Fcn104/1
  Transfer Fcn104/1 -> 2/1  "Vy"
  2/1 -> Sum66/4
  Constant24/1 -> Sum65/2
  Sum66/1 -> a2/1
  a2/1 -> Transfer Fcn99/1, Gain134/1  "P4"
  Transfer Fcn99/1 -> Sum65/3  "P5'"
  Gain134/1 -> Sum67/3
  Sum67/1 -> Transfer Fcn100/1
  Transfer Fcn100/1 -> Transfer Fcn102/1, Gain135/1
  Transfer Fcn102/1 -> Transfer Fcn101/1  "Vx'"
  Transfer Fcn101/1 -> Transfer Fcn105/1  "PA"
  Gain135/1 -> Sum66/7
  Transfer Fcn105/1 -> Sum67/1
  Constant25/1 -> Transfer Fcn106/1
  Transfer Fcn106/1 -> Sum67/2
  Sum68/1 -> Transfer Fcn109/1
  Transfer Fcn109/1 -> 3/1  "Vy"
  3/1 -> Sum69/4
  Constant26/1 -> Sum68/2
  Sum69/1 -> a4/1
  a4/1 -> Gain136/1, Transfer Fcn112/1  "P4"
  Transfer Fcn112/1 -> Sum68/3  "P5'"
  Gain136/1 -> Sum70/3
  Sum70/1 -> Transfer Fcn103/1
  Transfer Fcn103/1 -> Transfer Fcn108/1, Gain137/1
  Transfer Fcn108/1 -> Transfer Fcn107/1  "Vx'"
  Transfer Fcn107/1 -> Transfer Fcn110/1  "PA"
  Gain137/1 -> Sum69/7
  Transfer Fcn110/1 -> Sum70/1
  Constant27/1 -> Transfer Fcn111/1
  Transfer Fcn111/1 -> Sum70/2
  Sum71/1 -> Transfer Fcn116/1
  Transfer Fcn116/1 -> 4/1  "Vy"
  Constant28/1 -> Sum71/2
  4/1 -> a5/1
  a5/1 -> Gain138/1, Transfer Fcn119/1  "P4'"
  Transfer Fcn119/1 -> Sum71/3  "P5'"
  Gain138/1 -> Sum73/3
  Sum73/1 -> Transfer Fcn113/1
  Transfer Fcn113/1 -> Transfer Fcn120/1, Transfer Fcn115/1
  Transfer Fcn115/1 -> Transfer Fcn114/1  "Vx'"
  Transfer Fcn114/1 -> Transfer Fcn117/1  "PA"
  Transfer Fcn117/1 -> Sum73/1
  Constant29/1 -> Transfer Fcn118/1
  Transfer Fcn118/1 -> Sum73/2
  Transfer Fcn120/1 -> Transfer Fcn121/1
  Transfer Fcn121/1 -> Sum71/1
  Sum72/1 -> Transfer Fcn125/1
  Transfer Fcn125/1 -> 5/1  "Vy"
  Constant30/1 -> Sum72/2
  5/1 -> a6/1
  a6/1 -> Sum74/3, Transfer Fcn128/1  "P4"
  Transfer Fcn128/1 -> Sum72/3  "P5'"
  Transfer Fcn122/1 -> Transfer Fcn124/1, Transfer Fcn129/1
  Transfer Fcn124/1 -> Transfer Fcn123/1  "Vx'"
  Transfer Fcn123/1 -> Transfer Fcn126/1  "PA"
  Constant31/1 -> Transfer Fcn127/1
  Transfer Fcn129/1 -> Transfer Fcn130/1
  Transfer Fcn130/1 -> Sum72/1
  Transfer Fcn127/1 -> Sum74/1
  Transfer Fcn126/1 -> Gain139/1
  Sum74/1 -> Transfer Fcn122/1
  Gain139/1 -> Sum74/2
  Sum75/1 -> Transfer Fcn134/1
  Transfer Fcn134/1 -> 6/1  "Vy"
  Constant32/1 -> Sum75/2
  6/1 -> a7/1
  a7/1 -> Sum76/3, Transfer Fcn137/1  "P4"
  Transfer Fcn137/1 -> Sum75/3  "P5'"
  Transfer Fcn131/1 -> Transfer Fcn133/1, Transfer Fcn138/1
  Transfer Fcn133/1 -> Transfer Fcn132/1  "Vx'"
  Transfer Fcn132/1 -> Transfer Fcn135/1  "PA"
  Constant33/1 -> Transfer Fcn136/1
  Transfer Fcn138/1 -> Transfer Fcn139/1
  Transfer Fcn139/1 -> Sum75/1
  Transfer Fcn136/1 -> Sum76/1
  Transfer Fcn135/1 -> Gain140/1
  Sum76/1 -> Transfer Fcn131/1
  Gain140/1 -> Sum76/2
  Sum77/1 -> Transfer Fcn143/1
  Transfer Fcn143/1 -> 7/1  "Vy"
  Constant34/1 -> Sum77/2
  7/1 -> a8/1
  a8/1 -> Sum78/3, Transfer Fcn146/1  "P4"
  Transfer Fcn146/1 -> Sum77/3  "P5'"
  Transfer Fcn140/1 -> Transfer Fcn142/1, Transfer Fcn147/1
  Transfer Fcn142/1 -> Transfer Fcn141/1  "Vx'"
  Transfer Fcn141/1 -> Transfer Fcn144/1  "PA"
  Constant35/1 -> Transfer Fcn145/1
  Transfer Fcn147/1 -> Transfer Fcn148/1
  Transfer Fcn148/1 -> Sum77/1
  Transfer Fcn145/1 -> Sum78/1
  Transfer Fcn144/1 -> Gain141/1
  Sum78/1 -> Transfer Fcn140/1
  Gain141/1 -> Sum78/2
  Sum79/1 -> Transfer Fcn149/1
  Transfer Fcn149/1 -> Transfer Fcn150/1, Gain163/1, Gain162/1  "Vy"
  Gain142/1 -> Sum81/4, Sum80/4
  Constant36/1 -> Sum79/2
  Sum80/1 -> Tra/1
  Tra/1 -> Gain161/1, Gain144/1, Gain154/1  "P4"
  Sum81/1 -> Transfer Fcn152/1
  Transfer Fcn152/1 -> Gain146/1, Gain164/1, Gain145/1  "△P"
  Gain154/1 -> Sum82/3
  Sum82/1 -> Transfer Fcn153/1
  Transfer Fcn153/1 -> Gain192/1, Gain160/1, Gain148/1, Gain147/1, Gain156/1
  Gain156/1 -> Sum83/2
  Sum83/1 -> Transfer Fcn155/1
  Transfer Fcn155/1 -> Transfer Fcn156/1, Gain152/1, Gain158/1  "Vx"
  Transfer Fcn156/1 -> Gain157/1  "x"
  Gain157/1 -> Sum84/4
  Sum84/1 -> Transfer Fcn154/1
  Transfer Fcn154/1 -> Gain153/1, Gain260/1, Gain149/1, Gain151/1, Gain150/1  "PA"
  Gain160/1 -> Sum80/7
  Gain161/1 -> Sum80/1
  Gain162/1 -> Sum80/2
  Gain144/1 -> Sum80/3
  Gain147/1 -> Sum82/1
  Gain148/1 -> Sum82/2
  Gain149/1 -> Sum84/6
  Constant37/1 -> Sum83/1
  Gain150/1 -> Sum83/3
  Gain151/1 -> Sum84/5
  Gain152/1 -> Sum84/3
  Gain153/1 -> Sum84/2
  Gain158/1 -> Sum82/4
  Gain163/1 -> Sum81/1
  Gain164/1 -> Sum81/3
  Transfer Fcn150/1 -> Gain142/1  "y"
  Gain145/1 -> Sum80/6
  Gain146/1 -> Sum79/3
  Sum85/1 -> Transfer Fcn157/1
  Transfer Fcn157/1 -> Transfer Fcn158/1  "Vy"
  Gain165/1 -> Sum86/4
  Constant38/1 -> Sum85/2
  Sum86/1 -> Transfer Fcn159/1
  Transfer Fcn159/1 -> Gain183/1, Gain177/1  "P4"
  Transfer Fcn160/1 -> Gain168/1, Gain169/1  "△P"
  Gain177/1 -> Sum88/3
  Sum88/1 -> Transfer Fcn161/1
  Transfer Fcn161/1 -> Gain232/1, Gain170/1, Gain182/1, Gain178/1
  Gain178/1 -> Sum89/2
  Sum89/1 -> Transfer Fcn163/1
  Transfer Fcn163/1 -> Gain180/1, Gain175/1, Transfer Fcn164/1  "Vx"
  Transfer Fcn164/1 -> Gain179/1  "x"
  Gain179/1 -> Sum90/4
  Sum90/1 -> Transfer Fcn162/1
  Transfer Fcn162/1 -> Gain173/1, Gain172/1  "PA"
  Gain182/1 -> Sum86/7
  Gain183/1 -> Sum86/1
  Gain184/1 -> Sum86/2
  Gain170/1 -> Sum88/1
  Gain172/1 -> Sum90/6, Sum88/5
  Constant39/1 -> Sum89/1
  Gain173/1 -> Sum89/3
  Gain175/1 -> Sum90/3
  Gain180/1 -> Sum88/4
  Transfer Fcn158/1 -> Gain184/1, Transfer Fcn160/1, Gain165/1  "y"
  Gain168/1 -> Sum86/6
  Gain169/1 -> Sum85/3
  Sum87/1 -> Transfer Fcn165/1
  Transfer Fcn165/1 -> Transfer Fcn166/1  "Vy"
  Gain143/1 -> Sum91/4
  Constant40/1 -> Sum87/2
  Sum91/1 -> Transfer Fcn167/1
  Transfer Fcn167/1 -> Gain191/1, Gain185/1  "P4"
  Transfer Fcn168/1 -> Gain166/1  "△P"
  Gain185/1 -> Sum92/3
  Sum92/1 -> Transfer Fcn169/1
  Transfer Fcn169/1 -> Gain233/1, Gain167/1, Gain190/1, Gain186/1
  Gain186/1 -> Sum93/2
  Sum93/1 -> Transfer Fcn171/1
  Transfer Fcn171/1 -> Gain188/1, Gain176/1, Transfer Fcn172/1  "Vx"
  Transfer Fcn172/1 -> Gain187/1  "x"
  Gain187/1 -> Sum94/4
  Sum94/1 -> Transfer Fcn170/1
  Transfer Fcn170/1 -> Gain174/1, Gain171/1  "PA"
  Gain190/1 -> Sum91/7
  Gain191/1 -> Sum91/1
  Gain167/1 -> Sum92/1
  Gain171/1 -> Sum94/6, Sum92/5
  Gain174/1 -> Sum93/3
  Gain176/1 -> Sum94/3
  Gain188/1 -> Sum92/4
  Transfer Fcn166/1 -> Gain230/1, Gain143/1, Transfer Fcn173/1, Transfer Fcn168/1  "y"
  Gain155/1 -> Sum91/6
  Gain166/1 -> Sum87/3
  Transfer Fcn173/1 -> Gain155/1
  Sum100/1 -> Transfer Fcn183/1
  Transfer Fcn183/1 -> Transfer Fcn184/1  "Vy"
  Gain208/1 -> Sum101/4
  Constant44/1 -> Sum100/2
  Sum101/1 -> Transfer Fcn185/1
  Transfer Fcn185/1 -> Gain225/1, Gain209/1, Gain219/1  "P4"
  Sum102/1 -> Transfer Fcn186/1
  Transfer Fcn186/1 -> Gain210/1, Gain211/1, Gain228/1  "△P"
  Gain219/1 -> Sum103/3
  Sum103/1 -> Transfer Fcn187/1
  Transfer Fcn187/1 -> Gain231/1, Gain224/1, Gain213/1, Gain212/1, Gain220/1
  Gain220/1 -> Sum104/2
  Sum104/1 -> Transfer Fcn189/1
  Transfer Fcn189/1 -> Transfer Fcn190/1, Gain217/1, Gain222/1  "Vx"
  Transfer Fcn190/1 -> Gain221/1  "x"
  Gain221/1 -> Sum105/4
  Sum105/1 -> Transfer Fcn188/1
  Transfer Fcn188/1 -> Gain218/1, Gain214/1, Gain216/1, Gain215/1  "PA"
  Gain224/1 -> Sum101/7
  Gain225/1 -> Sum101/1
  Gain226/1 -> Sum101/2
  Gain209/1 -> Sum101/3
  Gain212/1 -> Sum103/1
  Gain213/1 -> Sum103/2
  Gain214/1 -> Sum103/5, Sum105/6
  Constant45/1 -> Sum104/1
  Gain215/1 -> Sum104/3
  Gain216/1 -> Sum105/5
  Gain217/1 -> Sum105/3
  Gain218/1 -> Sum105/2
  Gain222/1 -> Sum103/4
  Gain227/1 -> Sum102/1
  Gain228/1 -> Sum102/3
  Transfer Fcn184/1 -> Gain227/1, Gain226/1, Gain229/1, Gain208/1  "y"
  Gain210/1 -> Sum101/6
  Gain211/1 -> Sum100/3
  Gain229/1 -> Sum102/4
  Gain230/1 -> Sum91/2
  Gain192/1 -> Sum84/1
  Gain231/1 -> Sum105/1
  Gain232/1 -> Sum90/1
  Gain233/1 -> Sum94/1
  Sum95/1 -> Transfer Fcn174/1
  Gain193/1 -> Sum96/4
  Constant42/1 -> Sum95/2
  Sum96/1 -> Transfer Fcn176/1
  Transfer Fcn176/1 -> Gain206/1, Gain200/1  "P4"
  Gain200/1 -> Sum97/3
  Sum97/1 -> Transfer Fcn178/1
  Transfer Fcn178/1 -> Gain234/1, Gain196/1, Gain205/1, Gain201/1
  Gain201/1 -> Sum98/2
  Sum98/1 -> Transfer Fcn180/1
  Transfer Fcn180/1 -> Gain203/1, Gain199/1, Transfer Fcn181/1  "Vx"
  Transfer Fcn181/1 -> Gain202/1  "x"
  Gain202/1 -> Sum99/4
  Sum99/1 -> Transfer Fcn179/1
  Transfer Fcn179/1 -> Gain198/1, Gain197/1  "PA"
  Gain205/1 -> Sum96/7
  Gain206/1 -> Sum96/1
  Gain196/1 -> Sum97/1
  Gain197/1 -> Sum99/6, Sum97/5
  Constant43/1 -> Sum98/1
  Gain198/1 -> Sum98/3
  Gain199/1 -> Sum99/3
  Gain203/1 -> Sum97/4
  Transfer Fcn174/1 -> Gain207/1, Gain193/1, Transfer Fcn182/1  "y"
  Gain194/1 -> Sum96/6
  Transfer Fcn182/1 -> Gain194/1
  Gain207/1 -> Sum96/2
  Gain234/1 -> Sum99/1
  Sum106/1 -> Transfer Fcn175/1
  Transfer Fcn195/1 -> Sum107/1
  Constant46/1 -> Sum106/2
  Sum107/1 -> Transfer Fcn177/1
  Transfer Fcn177/1 -> Gain240/1  "P4"
  Gain240/1 -> Sum108/3
  Sum108/1 -> Transfer Fcn191/1
  Transfer Fcn191/1 -> Gain248/1, Gain236/1, Gain245/1, Gain241/1
  Gain241/1 -> Sum109/2
  Sum109/1 -> Transfer Fcn193/1
  Transfer Fcn193/1 -> Gain243/1, Gain239/1, Transfer Fcn194/1  "Vx"
  Transfer Fcn194/1 -> Gain242/1  "x"
  Gain242/1 -> Sum110/4
  Sum110/1 -> Transfer Fcn192/1
  Transfer Fcn192/1 -> Gain238/1, Gain237/1  "PA"
  Gain245/1 -> Sum107/2
  Gain236/1 -> Sum108/1
  Gain237/1 -> Sum110/6, Sum108/5
  Constant47/1 -> Sum109/1
  Gain238/1 -> Sum109/3
  Gain239/1 -> Sum110/3
  Gain243/1 -> Sum108/4
  Transfer Fcn175/1 -> Transfer Fcn195/1  "y"
  Gain248/1 -> Sum110/1
  Sum111/1 -> Transfer Fcn196/1
  Transfer Fcn202/1 -> Sum112/1
  Constant48/1 -> Sum111/2
  Sum112/1 -> Transfer Fcn197/1
  Transfer Fcn197/1 -> Gain249/1  "P4"
  Gain249/1 -> Sum113/3
  Sum113/1 -> Transfer Fcn203/1
  Transfer Fcn203/1 -> Gain255/1, Gain254/1, Gain250/1
  Gain250/1 -> Sum114/2
  Sum114/1 -> Transfer Fcn200/1
  Transfer Fcn200/1 -> Gain252/1, Gain247/1, Transfer Fcn201/1  "Vx"
  Transfer Fcn201/1 -> Gain251/1  "x"
  Gain251/1 -> Sum115/4
  Sum115/1 -> Transfer Fcn198/1
  Transfer Fcn198/1 -> Gain246/1, Gain258/1  "PA"
  Gain254/1 -> Sum112/2
  Gain246/1 -> Sum114/3
  Gain247/1 -> Sum115/3
  Gain252/1 -> Sum113/4
  Transfer Fcn196/1 -> Transfer Fcn202/1  "y"
  Gain255/1 -> Sum115/1
  Gain256/1 -> Sum3/5
  Gain258/1 -> Sum113/5
  Gain257/1 -> Sum5/1
  Gain259/1 -> Sum2/1
  Gain260/1 -> Sum82/5
  Sum116/1 -> 先导级/1
  Transfer Fcn208/1 -> Sum117/1
  Constant50/1 -> Sum116/2
  Sum117/1 -> Transfer Fcn204/1
  Transfer Fcn204/1 -> Gain261/1  "P4"
  Gain261/1 -> Sum118/3
  Sum118/1 -> Transfer Fcn209/1
  Transfer Fcn209/1 -> Gain266/1, 67/1, Gain262/1
  Gain262/1 -> Sum119/2
  Sum119/1 -> Transfer Fcn206/1
  Transfer Fcn206/1 -> Transfer Fcn207/1, Gain264/1  "Vx'"
  Transfer Fcn207/1 -> Sum120/4  "x'"
  Sum120/1 -> Transfer Fcn205/1
  Transfer Fcn205/1 -> 95/1, 68/1  "PA"
  Gain266/1 -> Sum117/2
  Gain264/1 -> Sum118/4
  先导级/1 -> Transfer Fcn208/1  "y"
  67/1 -> Sum120/1
  68/1 -> Sum118/5
  95/1 -> Sum119/3
  Sum121/1 -> 先导级1/1
  Transfer Fcn213/1 -> Sum122/1
  Constant51/1 -> Sum121/2
  Sum122/1 -> Transfer Fcn199/1
  Transfer Fcn199/1 -> Gain159/1  "P4"
  Gain159/1 -> Sum123/3
  Sum123/1 -> Transfer Fcn214/1
  Transfer Fcn214/1 -> 9/1, Gain195/1, Gain181/1
  Gain181/1 -> Sum124/2
  Sum124/1 -> Transfer Fcn211/1
  Transfer Fcn211/1 -> Sum126/2, Gain189/1  "Vx''"
  Transfer Fcn212/1 -> Sum125/4  "x'"
  Sum125/1 -> Transfer Fcn210/1
  Transfer Fcn210/1 -> Transfer Fcn216/1, Transfer Fcn215/1, 10/1  "PA"
  Gain195/1 -> Sum122/2
  Gain189/1 -> Sum123/4
  先导级1/1 -> Transfer Fcn213/1  "y"
  9/1 -> Sum125/1
  10/1 -> Sum123/5
  Sum126/1 -> Transfer Fcn212/1
  Transfer Fcn216/1 -> Sum123/6
  Sum127/1 -> 先导级2/1
  Transfer Fcn221/1 -> Sum128/1
  Constant52/1 -> Sum127/2
  Sum128/1 -> Transfer Fcn217/1
  Transfer Fcn217/1 -> Gain204/1  "P4"
  Gain204/1 -> Sum129/3
  Sum129/1 -> Transfer Fcn222/1
  Transfer Fcn222/1 -> 14/1, Gain244/1, Transfer Fcn219/1  "PB"
  Transfer Fcn219/1 -> Sum132/2, Gain235/1  "Vx''"
  Transfer Fcn220/1 -> Sum131/4  "x'"
  Sum131/1 -> Transfer Fcn218/1
  Transfer Fcn218/1 -> Transfer Fcn256/1, Transfer Fcn151/1  "PA"
  Gain244/1 -> Sum128/2
  Gain235/1 -> Sum129/4
  先导级2/1 -> Transfer Fcn221/1  "y"
  14/1 -> Sum131/1
  Sum132/1 -> Transfer Fcn220/1
  Transfer Fcn151/1 -> Sum129/6
  Sum130/1 -> 先导级3/1
  Constant53/1 -> Sum130/2
  Sum133/1 -> Transfer Fcn225/1
  Transfer Fcn225/1 -> Gain223/1  "P4"
  Gain223/1 -> Gain265/1, Sum134/3
  Sum134/1 -> Transfer Fcn230/1
  Transfer Fcn230/1 -> 15/1, Gain253/1
  Gain253/1 -> Sum135/2
  Sum135/1 -> Transfer Fcn227/1
  Transfer Fcn227/1 -> Transfer Fcn228/1, Transfer Fcn231/1, Gain263/1  "Vx'"
  Transfer Fcn228/1 -> Sum136/4  "x'"
  Sum136/1 -> Transfer Fcn226/1
  Transfer Fcn226/1 -> Transfer Fcn232/1, 17/1, 16/1  "PA"
  C3/1 -> Sum135/1
  Gain263/1 -> Sum134/4
  先导级3/1 -> Transfer Fcn229/1  "y"
  15/1 -> Sum136/1
  16/1 -> Sum134/5
  17/1 -> Sum135/3
  Transfer Fcn231/1 -> Sum133/3
  Transfer Fcn232/1 -> Sum133/4
  Transfer Fcn229/1 -> Sum133/2
  Gain265/1 -> Sum133/1
  Sum137/1 -> 先导级4/1
  Constant54/1 -> Sum137/2
  Sum138/1 -> Transfer Fcn233/1
  Transfer Fcn233/1 -> Gain267/1  "P4"
  Gain267/1 -> Gain270/1, Sum139/3
  Sum139/1 -> Transfer Fcn238/1
  Transfer Fcn238/1 -> 18/1, Gain268/1
  Gain268/1 -> Sum140/2
  Sum140/1 -> Transfer Fcn235/1
  Transfer Fcn235/1 -> Transfer Fcn236/1, Transfer Fcn239/1, Gain269/1  "Vx'"
  Transfer Fcn236/1 -> Sum141/4  "x'"
  Sum141/1 -> Transfer Fcn234/1
  Transfer Fcn234/1 -> Transfer Fcn240/1, 20/1, 19/1  "PA"
  C4/1 -> Sum140/1
  Gain269/1 -> Sum139/4
  先导级4/1 -> Transfer Fcn237/1  "y"
  18/1 -> Sum141/1
  19/1 -> Sum139/5
  20/1 -> Sum140/3
  Transfer Fcn239/1 -> Sum138/3
  Transfer Fcn240/1 -> Sum138/4
  Transfer Fcn237/1 -> Sum138/2
  Gain270/1 -> Sum138/1
  Sum142/1 -> 先导级5/1
  Transfer Fcn245/1 -> Sum143/1
  Constant55/1 -> Sum142/2
  Sum143/1 -> Transfer Fcn241/1
  Transfer Fcn241/1 -> Gain271/1  "P4"
  Gain271/1 -> Sum144/3
  Sum144/1 -> Transfer Fcn246/1
  Transfer Fcn246/1 -> Transfer Fcn243/1, Gain273/1
  Transfer Fcn243/1 -> Sum146/1, Gain272/1, Transfer Fcn249/1  "Vx''"
  Transfer Fcn244/1 -> Sum145/4  "x'"
  Sum145/1 -> Transfer Fcn242/1
  Transfer Fcn242/1 -> Transfer Fcn259/1, Transfer Fcn248/1, 21/1  "PA"
  Gain273/1 -> Sum143/2
  Gain272/1 -> Sum144/4
  先导级5/1 -> Transfer Fcn245/1  "y"
  23/1 -> Sum145/1
  21/1 -> Sum144/5
  Transfer Fcn248/1 -> Sum144/6
  Transfer Fcn249/1 -> 23/1
  Sum147/1 -> 先导级6/1
  Transfer Fcn254/1 -> Sum148/1
  Constant56/1 -> Sum147/2
  Sum148/1 -> Transfer Fcn250/1
  Transfer Fcn250/1 -> Gain274/1  "P4"
  Gain274/1 -> Sum149/3
  Sum149/1 -> Transfer Fcn255/1
  Transfer Fcn255/1 -> Transfer Fcn252/1, Gain276/1
  Transfer Fcn252/1 -> Sum151/1, Gain275/1  "Vx''"
  Transfer Fcn253/1 -> Sum150/4  "x'"
  Sum150/1 -> Transfer Fcn251/1
  Transfer Fcn251/1 -> Transfer Fcn260/1, Transfer Fcn257/1, 24/1, Transfer Fcn328/1  "PA"
  Gain276/1 -> Sum148/2
  Gain275/1 -> Sum149/4
  先导级6/1 -> Transfer Fcn254/1  "y"
  Transfer Fcn258/1 -> Sum150/1
  24/1 -> Sum149/5
  Transfer Fcn257/1 -> Sum149/6
  Sum152/1 -> 先导级7/1
  Transfer Fcn265/1 -> Sum153/1
  Constant57/1 -> Sum152/2
  Sum153/1 -> Transfer Fcn261/1
  Transfer Fcn261/1 -> Gain277/1  "P4"
  Gain277/1 -> Sum154/3
  Sum154/1 -> Transfer Fcn266/1
  Transfer Fcn266/1 -> Transfer Fcn263/1, Gain279/1
  Transfer Fcn263/1 -> Sum156/2, Gain278/1  "Vx''"
  Transfer Fcn264/1 -> Transfer Fcn262/1  "x''"
  Transfer Fcn262/1 -> Transfer Fcn327/1, Transfer Fcn268/1  "PA"
  Gain279/1 -> Sum153/2
  Gain278/1 -> Sum154/4
  先导级7/1 -> Transfer Fcn265/1  "y"
  Sum156/1 -> Transfer Fcn264/1
  Transfer Fcn268/1 -> Sum154/6
  Sum155/1 -> 先导级8/1
  Transfer Fcn270/1 -> Sum157/1
  Constant58/1 -> Sum155/2
  Sum157/1 -> Transfer Fcn223/1
  Transfer Fcn223/1 -> Gain280/1  "P4"
  Gain280/1 -> Sum158/3
  Sum158/1 -> Transfer Fcn271/1
  Transfer Fcn271/1 -> Transfer Fcn267/1
  Transfer Fcn267/1 -> Transfer Fcn273/1, Sum159/2, Gain281/1  "Vx''"
  Transfer Fcn269/1 -> Transfer Fcn247/1  "x'"
  Transfer Fcn247/1 -> Transfer Fcn272/1, Transfer Fcn329/1  "PA"
  Gain282/1 -> Sum157/2
  Gain281/1 -> Sum158/4
  先导级8/1 -> Transfer Fcn270/1  "y"
  Sum159/1 -> Transfer Fcn269/1
  Transfer Fcn272/1 -> Sum158/6
  Transfer Fcn273/1 -> Gain282/1
  Sum160/1 -> 先导级9/1
  Transfer Fcn278/1 -> Sum161/1
  Constant59/1 -> Sum160/2
  Sum161/1 -> Transfer Fcn274/1
  Transfer Fcn274/1 -> Gain283/1  "P4"
  Gain283/1 -> Sum162/3
  Sum162/1 -> Transfer Fcn279/1
  Transfer Fcn279/1 -> Transfer Fcn281/1, Sum163/2, Gain284/1  "Vx''"
  Transfer Fcn277/1 -> Transfer Fcn275/1  "x''"
  Transfer Fcn275/1 -> Transfer Fcn330/1, Transfer Fcn280/1  "PA"
  Transfer Fcn281/1 -> Sum161/2
  Gain284/1 -> Sum162/4
  先导级9/1 -> Transfer Fcn278/1  "y"
  Transfer Fcn330/1 -> Sum163/3
  Sum163/1 -> Transfer Fcn277/1
  Transfer Fcn280/1 -> Sum162/6
  Sum167/1 -> 先导级11/1
  Constant61/1 -> Sum167/2
  Transfer Fcn289/1 -> Transfer Fcn283/1
  Transfer Fcn283/1 -> Gain286/1  "P4"
  Gain286/1 -> Transfer Fcn293/1, Sum169/2
  Sum169/1 -> Transfer Fcn290/1
  Transfer Fcn290/1 -> Transfer Fcn288/1  "Vx'"
  Transfer Fcn288/1 -> Transfer Fcn291/1  "PA"
  Transfer Fcn291/1 -> Transfer Fcn295/1, Sum169/3
  Transfer Fcn293/1 -> Transfer Fcn292/1
  Transfer Fcn295/1 -> Transfer Fcn294/1
  先导级11/1 -> Sum173/2  "y"
  Sum173/1 -> Transfer Fcn289/1
  Transfer Fcn292/1 -> Transfer Fcn305/1
  Transfer Fcn305/1 -> Sum173/1
  Transfer Fcn294/1 -> Transfer Fcn306/1
  Transfer Fcn306/1 -> Sum173/3
  Sum168/1 -> 先导级12/1
  Constant62/1 -> Sum168/2
  Transfer Fcn298/1 -> Transfer Fcn296/1
  Transfer Fcn296/1 -> Gain287/1  "P4"
  Gain287/1 -> Transfer Fcn302/1, Sum170/2
  Sum170/1 -> Transfer Fcn299/1
  Transfer Fcn299/1 -> Transfer Fcn297/1  "Vx'"
  Transfer Fcn297/1 -> Transfer Fcn300/1  "PA"
  Transfer Fcn300/1 -> Transfer Fcn304/1, Sum170/3
  Transfer Fcn302/1 -> Transfer Fcn301/1
  Transfer Fcn304/1 -> Transfer Fcn303/1
  先导级12/1 -> Sum171/2  "y"
  Sum171/1 -> Transfer Fcn298/1
  Transfer Fcn301/1 -> Transfer Fcn307/1
  Transfer Fcn307/1 -> Sum171/1
  Transfer Fcn303/1 -> Transfer Fcn308/1
  Transfer Fcn308/1 -> Sum171/3
  Sum172/1 -> 先导级13/1
  Constant63/1 -> Sum172/2
  Transfer Fcn311/1 -> Transfer Fcn309/1
  Transfer Fcn309/1 -> Transfer Fcn315/1, Sum174/2  "P4'"
  Sum174/1 -> Transfer Fcn312/1
  Transfer Fcn312/1 -> Transfer Fcn310/1  "Vx'"
  Transfer Fcn310/1 -> Transfer Fcn313/1  "PA"
  Transfer Fcn313/1 -> Transfer Fcn317/1, Sum174/3
  Transfer Fcn315/1 -> Transfer Fcn314/1
  Transfer Fcn317/1 -> Transfer Fcn316/1
  先导级13/1 -> Sum175/2  "y"
  Sum175/1 -> Transfer Fcn311/1
  Transfer Fcn314/1 -> Transfer Fcn318/1
  Transfer Fcn318/1 -> Sum175/1
  Transfer Fcn316/1 -> Transfer Fcn319/1
  Transfer Fcn319/1 -> Sum175/3
  Sum176/1 -> 先导级14/1
  Constant64/1 -> Sum176/2
  Transfer Fcn321/1 -> Sum178/2  "P4'"
  Sum178/1 -> Transfer Fcn322/1
  Transfer Fcn322/1 -> Transfer Fcn320/1, T1/1  "Vx'"
  Transfer Fcn320/1 -> Transfer Fcn323/1  "PA"
  先导级14/1 -> Transfer Fcn321/1  "y"
  Transfer Fcn323/1 -> Sum178/3
  T1/1 -> Sum178/1
  Sum177/1 -> 先导级15/1
  Constant65/1 -> Sum177/2
  Transfer Fcn324/1 -> Sum179/2  "P4'"
  Sum179/1 -> Transfer Fcn325/1
  Transfer Fcn325/1 -> Transfer Fcn287/1  "Vx'"
  Transfer Fcn287/1 -> Transfer Fcn326/1  "PA"
  先导级15/1 -> Transfer Fcn324/1  "y"
  Transfer Fcn326/1 -> Sum179/3
  Transfer Fcn215/1 -> Sum126/3
  Transfer Fcn256/1 -> Sum132/3
  Sum146/1 -> Transfer Fcn244/1
  Transfer Fcn259/1 -> Sum146/2
  Sum151/1 -> Transfer Fcn253/1, Transfer Fcn258/1
  Transfer Fcn260/1 -> Sum151/2
  Transfer Fcn327/1 -> Sum156/3
  Transfer Fcn328/1 -> Sum150/3
  Transfer Fcn329/1 -> Sum159/3
  Sum164/1 -> 先导级10/1
  Transfer Fcn284/1 -> Sum165/1
  Constant41/1 -> Sum164/2
  Sum165/1 -> Transfer Fcn224/1
  Transfer Fcn224/1 -> Gain285/1  "P4"
  Gain285/1 -> Sum166/3
  Sum166/1 -> Transfer Fcn285/1
  Transfer Fcn285/1 -> Transfer Fcn331/1, Sum180/2, Gain288/1  "Vx''"
  Sum180/1 -> Transfer Fcn276/1
  Transfer Fcn276/1 -> Transfer Fcn332/1, Transfer Fcn286/1  "PA"
  Transfer Fcn331/1 -> Sum165/2
  Gain288/1 -> Sum166/4
  先导级10/1 -> Transfer Fcn284/1  "y"
  Transfer Fcn332/1 -> Sum180/3
  Transfer Fcn286/1 -> Sum166/6
